simulink model "EPT"  (R2019b)
settings: Solver=FixedStepDiscrete  StartTime=0.0  StopTime=5  FixedStep=0.005  RelTol=1e-3  EnableMultiTasking=on
PreLoadFcn:
  | try, model_open; catch, disp('Error occurred while executing model pre-load callback: model_open.m'); disp('Please assure that the MATLAB working directory is set to the model directory before opening.'); end
InitFcn:
  | try, model_open; catch, end
undefined symbols (not defined in the file or in its folder): Bridge, GCM, H, ln, raptor_get_param_eval, raptor_get_safe_string, raptor_xcp_function
libraries: Raptor_lib x2810, simulink x374, hdlsllib x19
(part 8 of 45)

== system EPT/Test/LifeCycleTest/RollingCount1 ==
  In1 : Inport
  Add : Sum
  Constant3 : Constant
  Data Type Conversion : DataTypeConversion
  Data Type Conversion21 : DataTypeConversion
  NOT : Logic  Operator=NOT  IconShape=distinctive  AllPortsSameDT=off  OutDataTypeStr=boolean
  Relational Operator : RelationalOperator  Operator=>  OutDataTypeStr=boolean  RndMeth=Simplest
  Switch : Switch  Criteria=u2 > Threshold
  Unit Delay : UnitDelay  SampleTime=-1  HasFrameUpgradeWarning=on
  Out1 : Outport  VectorParamsAs1DForOutWhenUnconnected=off
  wires:
  Data Type Conversion/1 -> Out1/1
  NOT/1 -> Data Type Conversion21/1, Switch/3
  Unit Delay/1 -> Add/1
  Constant3/1 -> Add/2
  Relational Operator/1 -> NOT/1
  Add/1 -> Switch/1, Relational Operator/1
  Data Type Conversion21/1 -> Switch/2
  Switch/1 -> Data Type Conversion/1, Unit Delay/1
  In1/1 -> Relational Operator/2

== system EPT/Test/RPB1600_Read/CountTrigger ==
  Counter : Inport
  Constant1 : Constant  Value=0
  Constant3 : Constant
  CycleTrigger : Subsystem
  Switch : Switch  Threshold=1
  Unit Delay1 : UnitDelay  SampleTime=-1  HasFrameUpgradeWarning=on
  Unit Delay2 : UnitDelay  SampleTime=-1  HasFrameUpgradeWarning=on
  Tirgger : Outport  VectorParamsAs1DForOutWhenUnconnected=off
  wires:
  Unit Delay2/1 -> Tirgger/1
  Unit Delay1/1 -> CycleTrigger/1(In1)
  CycleTrigger/1(Trigger) -> Unit Delay2/1, Switch/2
  Counter/1 -> CycleTrigger/2(In2)
  Constant1/1 -> Switch/1
  Constant3/1 -> Switch/3
  Switch/1 -> Unit Delay1/1

== system EPT/Test/RPB1600_Read/RPB1600_Cmd_20ms ==
  ID : Inport
  DataBytes : Inport  Port=2
  Command : Inport  Port=3
  Trigger : TriggerPort  VariantControl=Variant  PortDimensions=1
  Add : Sum
  Constant : Constant  Value=2
  Constant1 : Constant  OutDataTypeStr=boolean
  raptor_can_txraw : Raptor_lib/CAN/raptor_can_txraw  canBus='CAN1'  queueSize=1  showIdTypePort=1  idTypeSelectValues=Standard|Extended  idTypeSelect=Standard
      settings: SourceProductName=Raptor
  wires:
  Add/1 -> raptor_can_txraw/3
  DataBytes/1 -> Add/1
  Constant/1 -> Add/2
  Constant1/1 -> raptor_can_txraw/1
  Command/1 -> raptor_can_txraw/4
  ID/1 -> raptor_can_txraw/2

== system EPT/Test/RPB1600_Read/RPB1600_RX_20ms ==
  note: 0x0000:OPERATION
      | 0x0020:VOUT_SET
      | 0x0030:IOUT_SET
      | 0x0040:FAULT_STATUS
      | 0x0050:READ_VIN
      | 0x0060:READ_VOUT
      | 0x0061:READ_IOUT
      | 0x0062:READ_TEMPERATURE_1
      | 0x0070:READ_FAN_SPEED_1
      | 0x0071:READ_FAN_SPEED_2
  Task : Inport
  "Resolution " : Inport  Port=2
  Trigger : TriggerPort  TriggerType=falling  VariantControl=Variant  PortDimensions=1
  Constant : Constant  Value=0
  Constant1 : Constant
  Constant2 : Constant  Value=2
  Constant3 : Constant  Value=3
  Constant4 : Constant  Value=4
  Constant5 : Constant  Value=5
  Constant6 : Constant  Value=6
  Constant7 : Constant  Value=7
  Constant8 : Constant  Value=8
  Constant9 : Constant  Value=9
  Convert_Byte2Data : Subsystem
  Demux : Demux  Outputs=8
  Subsystem : Subsystem
  Subsystem1 : Subsystem
  Subsystem2 : Subsystem
  Subsystem3 : Subsystem
  Subsystem4 : Subsystem
  Subsystem5 : Subsystem
  Subsystem6 : Subsystem
  Subsystem7 : Subsystem
  Subsystem8 : Subsystem
  Subsystem9 : Subsystem
  Task Rolling : Subsystem
  raptor_can_rxraw : Raptor_lib/CAN/raptor_can_rxraw  canBus='CAN1'  extendedId=1  showAge=1  id=hex2dec('C0100')  idMask=hex2dec('1FFFFFFF')  mailbox=''  queueSize=1
      settings: SourceProductName=Raptor
  raptor_measurement : Raptor_lib/Data Storage/raptor_measurement  paramName='Read_OPERATION'  nameSource=Parameter  calDispType=Number  calEnum={'False', 'True'}  calGain=1.0  calOffset=0.0  calMax=inf  calMin=-inf  calFormat='-1'  calUnit=''  calHelp=''  calAccess=1  calFunction=raptor_xcp_function(gcb)  calVisible=on
      settings: SourceProductName=Raptor
  raptor_measurement1 : Raptor_lib/Data Storage/raptor_measurement  paramName='Read_VOUT_SET'  nameSource=Parameter  calDispType=Number  calEnum={'False', 'True'}  calGain=1.0  calOffset=0.0  calMax=inf  calMin=-inf  calFormat='-1'  calUnit=''  calHelp=''  calAccess=1  calFunction=raptor_xcp_function(gcb)  calVisible=on
      settings: SourceProductName=Raptor
  raptor_measurement2 : Raptor_lib/Data Storage/raptor_measurement  paramName='Read_IOUT_SET'  nameSource=Parameter  calDispType=Number  calEnum={'False', 'True'}  calGain=1.0  calOffset=0.0  calMax=inf  calMin=-inf  calFormat='-1'  calUnit=''  calHelp=''  calAccess=1  calFunction=raptor_xcp_function(gcb)  calVisible=on
      settings: SourceProductName=Raptor
  raptor_measurement3 : Raptor_lib/Data Storage/raptor_measurement  paramName='FAULT_STATUS'  nameSource=Parameter  calDispType=Number  calEnum={'False', 'True'}  calGain=1.0  calOffset=0.0  calMax=inf  calMin=-inf  calFormat='-1'  calUnit=''  calHelp=''  calAccess=1  calFunction=raptor_xcp_function(gcb)  calVisible=on
      settings: SourceProductName=Raptor
  raptor_measurement4 : Raptor_lib/Data Storage/raptor_measurement  paramName='READ_VIN'  nameSource=Parameter  calDispType=Number  calEnum={'False', 'True'}  calGain=1.0  calOffset=0.0  calMax=inf  calMin=-inf  calFormat='-1'  calUnit=''  calHelp=''  calAccess=1  calFunction=raptor_xcp_function(gcb)  calVisible=on
      settings: SourceProductName=Raptor
  raptor_measurement5 : Raptor_lib/Data Storage/raptor_measurement  paramName='READ_VOUT'  nameSource=Parameter  calDispType=Number  calEnum={'False', 'True'}  calGain=1.0  calOffset=0.0  calMax=inf  calMin=-inf  calFormat='-1'  calUnit=''  calHelp=''  calAccess=1  calFunction=raptor_xcp_function(gcb)  calVisible=on
      settings: SourceProductName=Raptor
  raptor_measurement6 : Raptor_lib/Data Storage/raptor_measurement  paramName='READ_TEMPERATURE_1'  nameSource=Parameter  calDispType=Number  calEnum={'False', 'True'}  calGain=1.0  calOffset=0.0  calMax=inf  calMin=-inf  calFormat='-1'  calUnit=''  calHelp=''  calAccess=1  calFunction=raptor_xcp_function(gcb)  calVisible=on
      settings: SourceProductName=Raptor
  raptor_measurement7 : Raptor_lib/Data Storage/raptor_measurement  paramName='READ_IOUT'  nameSource=Parameter  calDispType=Number  calEnum={'False', 'True'}  calGain=1.0  calOffset=0.0  calMax=inf  calMin=-inf  calFormat='-1'  calUnit=''  calHelp=''  calAccess=1  calFunction=raptor_xcp_function(gcb)  calVisible=on
      settings: SourceProductName=Raptor
  raptor_measurement8 : Raptor_lib/Data Storage/raptor_measurement  paramName='READ_FAN_SPEED_1'  nameSource=Parameter  calDispType=Number  calEnum={'False', 'True'}  calGain=1.0  calOffset=0.0  calMax=inf  calMin=-inf  calFormat='-1'  calUnit=''  calHelp=''  calAccess=1  calFunction=raptor_xcp_function(gcb)  calVisible=on
      settings: SourceProductName=Raptor
  raptor_measurement9 : Raptor_lib/Data Storage/raptor_measurement  paramName='READ_FAN_SPEED_2'  nameSource=Parameter  calDispType=Number  calEnum={'False', 'True'}  calGain=1.0  calOffset=0.0  calMax=inf  calMin=-inf  calFormat='-1'  calUnit=''  calHelp=''  calAccess=1  calFunction=raptor_xcp_function(gcb)  calVisible=on
      settings: SourceProductName=Raptor
  wires:
  Task/1 -> Subsystem7/2(Task Input), Subsystem8/2(Task Input), Subsystem9/2(Task Input), Subsystem6/2(Task Input), Subsystem5/2(Task Input), Subsystem4/2(Task Input), Subsystem3/2(Task Input), Subsystem2/2(Task Input), Subsystem1/2(Task Input), Subsystem/2(Task Input)
  Constant/1 -> Subsystem/3("Task Set ")
  Constant1/1 -> Subsystem1/3("Task Set ")
  Constant2/1 -> Subsystem2/3("Task Set ")
  Constant4/1 -> Subsystem4/3("Task Set ")
  Constant5/1 -> Subsystem5/3("Task Set ")
  Constant6/1 -> Subsystem6/3("Task Set ")
  Constant7/1 -> Subsystem7/3("Task Set ")
  Constant9/1 -> Subsystem9/3("Task Set ")
  raptor_can_rxraw/5 -> Demux/1
  Demux/1 -> Convert_Byte2Data/1(LowByte)
  Demux/2 -> Convert_Byte2Data/2(HighByte)
  "Resolution "/1 -> Convert_Byte2Data/4(Factor)
  Constant3/1 -> Subsystem3/3("Task Set ")
  Constant8/1 -> Subsystem8/3("Task Set ")
  Convert_Byte2Data/1(Data(int16)) -> Subsystem9/1(Rx Data), Subsystem8/1(Rx Data), Subsystem7/1(Rx Data), Subsystem6/1(Rx Data), Subsystem5/1(Rx Data), Subsystem4/1(Rx Data), Subsystem3/1(Rx Data), Subsystem2/1(Rx Data), Subsystem1/1(Rx Data), Subsystem/1(Rx Data)
  Subsystem/1(Output) -> raptor_measurement/1
  Subsystem1/1(Output) -> raptor_measurement1/1
  Subsystem2/1(Output) -> raptor_measurement2/1
  Subsystem3/1(Output) -> raptor_measurement3/1
  Subsystem4/1(Output) -> raptor_measurement4/1
  Subsystem5/1(Output) -> raptor_measurement5/1
  Subsystem6/1(Output) -> raptor_measurement7/1
  Subsystem7/1(Output) -> raptor_measurement6/1
  Subsystem8/1(Output) -> raptor_measurement8/1
  Subsystem9/1(Output) -> raptor_measurement9/1

== system EPT/Foreground_TimeBase_5ms/CAN/CAN1_exec/BCU vs RMDA-BMS ==
  Trigger : TriggerPort  VariantControl=Variant  PortDimensions=1
  "BCU-OBU Output-CTL " : Subsystem
  BCU-OBU Output-EW Code : Subsystem
  BCU-OBU Status-OP G1 : Subsystem
  BCU-OBU Status-OP G2 : Subsystem
  BCU-OBU Status-OP G3 : Subsystem
  "BCU-OBU Status-OP G4 " : Subsystem
  "BP-OBU Enable CTL & OP Status " : Subsystem
  Compare To Constant : simulink/Logic and Bit Operations/Compare To Constant  relop===  const=0  OutDataTypeStr=boolean
  Compare To Constant1 : simulink/Logic and Bit Operations/Compare To Constant  relop===  const=10  OutDataTypeStr=boolean
  Compare To Constant2 : simulink/Logic and Bit Operations/Compare To Constant  relop===  const=20  OutDataTypeStr=boolean
  Compare To Constant3 : simulink/Logic and Bit Operations/Compare To Constant  relop===  const=30  OutDataTypeStr=boolean
  Compare To Constant4 : simulink/Logic and Bit Operations/Compare To Constant  relop===  const=40  OutDataTypeStr=boolean
  Compare To Constant5 : simulink/Logic and Bit Operations/Compare To Constant  relop===  const=50  OutDataTypeStr=boolean
  Compare To Constant6 : simulink/Logic and Bit Operations/Compare To Constant  relop===  const=60  OutDataTypeStr=boolean
  Compare To Constant7 : simulink/Logic and Bit Operations/Compare To Constant  relop===  const=70  OutDataTypeStr=boolean
  Compare To Constant8 : simulink/Logic and Bit Operations/Compare To Constant  relop===  const=80  OutDataTypeStr=boolean
  Compare To Constant9 : simulink/Logic and Bit Operations/Compare To Constant  relop===  const=90  OutDataTypeStr=boolean
  Constant2 : Constant  Value=100
  Constant3 : Constant  Value=100
  Delay{,1..8} (9 alike) : Delay
  Rem : Math  Operator=rem  SaturateOnIntegerOverflow=on
  Remote DAG2-5E0 : Subsystem
  Remote DAG2-5E1 : Subsystem
  Remote DAG2-5E2 : Subsystem
  Remote DAG2-5E3 : Subsystem
  Remote DAG2-5E4 : Subsystem
  Remote DAG2-5E5 : Subsystem
  Remote DAG2-5E6 : Subsystem
  Remote DAG2-5E7 : Subsystem
  Remote DAG2-5E8 : Subsystem
  Remote DAG2-5E9 : Subsystem
  Remote DAG2-5EA : Subsystem
  Remote DAG2-5EB : Subsystem
  RollingCount : Subsystem
  wires:
  Rem/1 -> Compare To Constant9/1, Compare To Constant8/1, Compare To Constant7/1, Compare To Constant6/1, Compare To Constant5/1, Compare To Constant4/1, Compare To Constant3/1, Compare To Constant2/1, Compare To Constant1/1, Compare To Constant/1
  Constant2/1 -> RollingCount/1(In1)
  Constant3/1 -> Rem/2
  RollingCount/1(Out1) -> Rem/1
  Compare To Constant9/1 -> Delay2/1, "BCU-OBU Status-OP G4 "/Trigger
  Compare To Constant8/1 -> BCU-OBU Status-OP G3/Trigger, Delay8/1
  Compare To Constant7/1 -> Delay7/1, BCU-OBU Status-OP G2/Trigger
  Compare To Constant6/1 -> Delay6/1, BCU-OBU Status-OP G1/Trigger
  Compare To Constant5/1 -> Delay4/1, "BCU-OBU Output-CTL "/Trigger
  Compare To Constant/1 -> Delay/1, Remote DAG2-5E0/Trigger
  Compare To Constant1/1 -> Delay1/1, Remote DAG2-5E1/Trigger
  Compare To Constant2/1 -> Delay3/1, Remote DAG2-5E2/Trigger
  Compare To Constant3/1 -> Remote DAG2-5E3/Trigger
  Compare To Constant4/1 -> Delay5/1, Remote DAG2-5E4/Trigger
  Delay/1 -> Remote DAG2-5E9/Trigger
  Delay1/1 -> Remote DAG2-5EA/Trigger
  Delay6/1 -> Remote DAG2-5E5/Trigger
  Delay7/1 -> Remote DAG2-5E6/Trigger
  Delay8/1 -> Remote DAG2-5E7/Trigger
  Delay2/1 -> Remote DAG2-5E8/Trigger
  Delay3/1 -> Remote DAG2-5EB/Trigger
  Delay4/1 -> BCU-OBU Output-EW Code/Trigger
  Delay5/1 -> "BP-OBU Enable CTL & OP Status "/Trigger

== system EPT/Foreground_TimeBase_5ms/CAN/CAN1_exec/BCU-CMU ==
  Enable : EnablePort
  CMU_Task : Subsystem

== system EPT/Foreground_TimeBase_5ms/CAN/CAN1_exec/CountTrigger1 ==
  Counter : Inport
  Constant1 : Constant  Value=0
  Constant3 : Constant
  CycleTrigger : Subsystem
  Switch : Switch  Threshold=1
  Unit Delay1 : UnitDelay  SampleTime=-1  HasFrameUpgradeWarning=on
  Unit Delay2 : UnitDelay  SampleTime=-1  HasFrameUpgradeWarning=on
  Tirgger : Outport  VectorParamsAs1DForOutWhenUnconnected=off
  wires:
  Switch/1 -> Unit Delay1/1
  Constant3/1 -> Switch/3
  Constant1/1 -> Switch/1
  Counter/1 -> CycleTrigger/2(In2)
  CycleTrigger/1(Trigger) -> Switch/2, Unit Delay2/1
  Unit Delay1/1 -> CycleTrigger/1(In1)
  Unit Delay2/1 -> Tirgger/1

== system EPT/Foreground_TimeBase_5ms/CAN/CAN1_exec/IVT ==
  Enable : EnablePort
  Constant1 : Constant  Value=4
  Constant2 : Constant  Value=12
  CountTrigger : Subsystem
  CountTrigger1 : Subsystem
  Delay : Delay  DelayLength=1
  "IVT_RX_0x521 " : Subsystem  TreatAsAtomicUnit=on
  IVT_RX_0x522 : Subsystem  TreatAsAtomicUnit=on
  IVT_RX_0x523 : Subsystem  TreatAsAtomicUnit=on
  IVT_RX_0x524 : Subsystem  TreatAsAtomicUnit=on
  wires:
  Delay/1 -> IVT_RX_0x523/Trigger, IVT_RX_0x524/Trigger
  Constant2/1 -> CountTrigger1/1(Counter)
  CountTrigger1/1(Tirgger) -> IVT_RX_0x522/Trigger, Delay/1
  CountTrigger/1(Tirgger) -> "IVT_RX_0x521 "/Trigger
  Constant1/1 -> CountTrigger/1(Counter)

== system EPT/Foreground_TimeBase_5ms/CAN/CAN2_exec/BCU vs ITRI//ARTC ==
  Enable : EnablePort
  "BCU-OBU Output-CTL " : Subsystem
  BCU-OBU Output-EW Code : Subsystem
  BCU-OBU Status-OP G1 : Subsystem
  BCU-OBU Status-OP G2 : Subsystem
  BCU-OBU Status-OP G3 : Subsystem
  "BCU-OBU Status-OP G4 " : Subsystem
  "BP-OBU Enable CTL & OP Status " : Subsystem
  CountTrigger1 : Subsystem
  Delay{,1..17} (18 alike) : Delay  DelayLength=1  InitialCondition=0  UseCircularBuffer=on
  Remote DAG2-5E0 : Subsystem
  Remote DAG2-5E1 : Subsystem
  Remote DAG2-5E2 : Subsystem
  Remote DAG2-5E3 : Subsystem
  Remote DAG2-5E4 : Subsystem
  Remote DAG2-5E5 : Subsystem
  Remote DAG2-5E6 : Subsystem
  Remote DAG2-5E7 : Subsystem
  Remote DAG2-5E8 : Subsystem
  Remote DAG2-5E9 : Subsystem
  Remote DAG2-5EA : Subsystem
  Remote DAG2-5EB : Subsystem
  raptor_adjustment : Raptor_lib/Data Storage/raptor_adjustment  paramName='Cal_CAN2ITRI_TxTime'  nameSource=Parameter  initValue=100  dataType=double  storage=Calibration  calDispType=Number  calEnum={'False', 'True'}  calGain=1.0  calOffset=0.0  calMax=inf  calMin=-inf  calFormat='-1'  calUnit=''  calHelp=''  calAccess=1  calFunction=raptor_xcp_function(gcb)  calDispHeaders=off  calColHeaders={'Col1' 'Col2' 'Col3'}  calRowHeaders={'Row1' 'Row2' 'Row3'}
      settings: SourceProductName=Raptor
  raptor_adjustment1 : Raptor_lib/Data Storage/raptor_adjustment  paramName='Cal_BCU_OBU_Status_OP_G1_CANon'  nameSource=Parameter  initValue=0.00  dataType=double  storage=Calibration  calDispType=Number  calEnum={'False', 'True'}  calGain=1.0  calOffset=0.0  calMax=inf  calMin=-inf  calFormat='-1'  calUnit=''  calHelp=''  calAccess=1  calFunction=raptor_xcp_function(gcb)  calDispHeaders=off  calColHeaders={'Col1' 'Col2' 'Col3'}  calRowHeaders={'Row1' 'Row2' 'Row3'}
      settings: SourceProductName=Raptor
  raptor_adjustment10 : Raptor_lib/Data Storage/raptor_adjustment  paramName='Cal_BCU_OBU_DAG2_5E7_CANon'  nameSource=Parameter  initValue=0.00  dataType=double  storage=Calibration  calDispType=Number  calEnum={'False', 'True'}  calGain=1.0  calOffset=0.0  calMax=inf  calMin=-inf  calFormat='-1'  calUnit=''  calHelp=''  calAccess=1  calFunction=raptor_xcp_function(gcb)  calDispHeaders=off  calColHeaders={'Col1' 'Col2' 'Col3'}  calRowHeaders={'Row1' 'Row2' 'Row3'}
      settings: SourceProductName=Raptor
  raptor_adjustment11 : Raptor_lib/Data Storage/raptor_adjustment  paramName='Cal_BCU_OBU_DAG2_5E8_CANon'  nameSource=Parameter  initValue=0.00  dataType=double  storage=Calibration  calDispType=Number  calEnum={'False', 'True'}  calGain=1.0  calOffset=0.0  calMax=inf  calMin=-inf  calFormat='-1'  calUnit=''  calHelp=''  calAccess=1  calFunction=raptor_xcp_function(gcb)  calDispHeaders=off  calColHeaders={'Col1' 'Col2' 'Col3'}  calRowHeaders={'Row1' 'Row2' 'Row3'}
      settings: SourceProductName=Raptor
  raptor_adjustment12 : Raptor_lib/Data Storage/raptor_adjustment  paramName='Cal_BCU_OBU_DAG2_5EB_CANon'  nameSource=Parameter  initValue=0.00  dataType=double  storage=Calibration  calDispType=Number  calEnum={'False', 'True'}  calGain=1.0  calOffset=0.0  calMax=inf  calMin=-inf  calFormat='-1'  calUnit=''  calHelp=''  calAccess=1  calFunction=raptor_xcp_function(gcb)  calDispHeaders=off  calColHeaders={'Col1' 'Col2' 'Col3'}  calRowHeaders={'Row1' 'Row2' 'Row3'}
      settings: SourceProductName=Raptor
  raptor_adjustment13 : Raptor_lib/Data Storage/raptor_adjustment  paramName='Cal_BCU_OBU_DAG2_5E9_CANon'  nameSource=Parameter  initValue=0.00  dataType=double  storage=Calibration  calDispType=Number  calEnum={'False', 'True'}  calGain=1.0  calOffset=0.0  calMax=inf  calMin=-inf  calFormat='-1'  calUnit=''  calHelp=''  calAccess=1  calFunction=raptor_xcp_function(gcb)  calDispHeaders=off  calColHeaders={'Col1' 'Col2' 'Col3'}  calRowHeaders={'Row1' 'Row2' 'Row3'}
      settings: SourceProductName=Raptor
  raptor_adjustment14 : Raptor_lib/Data Storage/raptor_adjustment  paramName='Cal_BCU_OBU_DAG2_5EA_CANon'  nameSource=Parameter  initValue=0.00  dataType=double  storage=Calibration  calDispType=Number  calEnum={'False', 'True'}  calGain=1.0  calOffset=0.0  calMax=inf  calMin=-inf  calFormat='-1'  calUnit=''  calHelp=''  calAccess=1  calFunction=raptor_xcp_function(gcb)  calDispHeaders=off  calColHeaders={'Col1' 'Col2' 'Col3'}  calRowHeaders={'Row1' 'Row2' 'Row3'}
      settings: SourceProductName=Raptor
  raptor_adjustment15 : Raptor_lib/Data Storage/raptor_adjustment  paramName='Cal_BCU_OBU_DAG2_5E3_CANon'  nameSource=Parameter  initValue=0.00  dataType=double  storage=Calibration  calDispType=Number  calEnum={'False', 'True'}  calGain=1.0  calOffset=0.0  calMax=inf  calMin=-inf  calFormat='-1'  calUnit=''  calHelp=''  calAccess=1  calFunction=raptor_xcp_function(gcb)  calDispHeaders=off  calColHeaders={'Col1' 'Col2' 'Col3'}  calRowHeaders={'Row1' 'Row2' 'Row3'}
      settings: SourceProductName=Raptor
  raptor_adjustment16 : Raptor_lib/Data Storage/raptor_adjustment  paramName='Cal_BCU_OBU_DAG2_5E4_CANon'  nameSource=Parameter  initValue=0.00  dataType=double  storage=Calibration  calDispType=Number  calEnum={'False', 'True'}  calGain=1.0  calOffset=0.0  calMax=inf  calMin=-inf  calFormat='-1'  calUnit=''  calHelp=''  calAccess=1  calFunction=raptor_xcp_function(gcb)  calDispHeaders=off  calColHeaders={'Col1' 'Col2' 'Col3'}  calRowHeaders={'Row1' 'Row2' 'Row3'}
      settings: SourceProductName=Raptor
  raptor_adjustment17 : Raptor_lib/Data Storage/raptor_adjustment  paramName='Cal_BCU_OBU_DAG2_5E0_CANon'  nameSource=Parameter  initValue=0.00  dataType=double  storage=Calibration  calDispType=Number  calEnum={'False', 'True'}  calGain=1.0  calOffset=0.0  calMax=inf  calMin=-inf  calFormat='-1'  calUnit=''  calHelp=''  calAccess=1  calFunction=raptor_xcp_function(gcb)  calDispHeaders=off  calColHeaders={'Col1' 'Col2' 'Col3'}  calRowHeaders={'Row1' 'Row2' 'Row3'}
      settings: SourceProductName=Raptor
  raptor_adjustment2 : Raptor_lib/Data Storage/raptor_adjustment  paramName='Cal_BCU_OBU_Status_OP_G2_CANon'  nameSource=Parameter  initValue=0.00  dataType=double  storage=Calibration  calDispType=Number  calEnum={'False', 'True'}  calGain=1.0  calOffset=0.0  calMax=inf  calMin=-inf  calFormat='-1'  calUnit=''  calHelp=''  calAccess=1  calFunction=raptor_xcp_function(gcb)  calDispHeaders=off  calColHeaders={'Col1' 'Col2' 'Col3'}  calRowHeaders={'Row1' 'Row2' 'Row3'}
      settings: SourceProductName=Raptor
  raptor_adjustment20 : Raptor_lib/Data Storage/raptor_adjustment  paramName='Cal_BCU_OBU_DAG2_5E1_CANon'  nameSource=Parameter  initValue=0.00  dataType=double  storage=Calibration  calDispType=Number  calEnum={'False', 'True'}  calGain=1.0  calOffset=0.0  calMax=inf  calMin=-inf  calFormat='-1'  calUnit=''  calHelp=''  calAccess=1  calFunction=raptor_xcp_function(gcb)  calDispHeaders=off  calColHeaders={'Col1' 'Col2' 'Col3'}  calRowHeaders={'Row1' 'Row2' 'Row3'}
      settings: SourceProductName=Raptor
  raptor_adjustment21 : Raptor_lib/Data Storage/raptor_adjustment  paramName='Cal_BCU_OBU_DAG2_5E2_CANon'  nameSource=Parameter  initValue=0.00  dataType=double  storage=Calibration  calDispType=Number  calEnum={'False', 'True'}  calGain=1.0  calOffset=0.0  calMax=inf  calMin=-inf  calFormat='-1'  calUnit=''  calHelp=''  calAccess=1  calFunction=raptor_xcp_function(gcb)  calDispHeaders=off  calColHeaders={'Col1' 'Col2' 'Col3'}  calRowHeaders={'Row1' 'Row2' 'Row3'}
      settings: SourceProductName=Raptor
  raptor_adjustment3 : Raptor_lib/Data Storage/raptor_adjustment  paramName='Cal_BCU_OBU_Status_OP_G3_CANon'  nameSource=Parameter  initValue=0.00  dataType=double  storage=Calibration  calDispType=Number  calEnum={'False', 'True'}  calGain=1.0  calOffset=0.0  calMax=inf  calMin=-inf  calFormat='-1'  calUnit=''  calHelp=''  calAccess=1  calFunction=raptor_xcp_function(gcb)  calDispHeaders=off  calColHeaders={'Col1' 'Col2' 'Col3'}  calRowHeaders={'Row1' 'Row2' 'Row3'}
      settings: SourceProductName=Raptor
  raptor_adjustment4 : Raptor_lib/Data Storage/raptor_adjustment  paramName='Cal_BCU_OBU_Status_OP_G4_CANon'  nameSource=Parameter  initValue=0.00  dataType=double  storage=Calibration  calDispType=Number  calEnum={'False', 'True'}  calGain=1.0  calOffset=0.0  calMax=inf  calMin=-inf  calFormat='-1'  calUnit=''  calHelp=''  calAccess=1  calFunction=raptor_xcp_function(gcb)  calDispHeaders=off  calColHeaders={'Col1' 'Col2' 'Col3'}  calRowHeaders={'Row1' 'Row2' 'Row3'}
      settings: SourceProductName=Raptor
  raptor_adjustment5 : Raptor_lib/Data Storage/raptor_adjustment  paramName='Cal_BCU_OBU_Output_CTL_CANon'  nameSource=Parameter  initValue=0.00  dataType=double  storage=Calibration  calDispType=Number  calEnum={'False', 'True'}  calGain=1.0  calOffset=0.0  calMax=inf  calMin=-inf  calFormat='-1'  calUnit=''  calHelp=''  calAccess=1  calFunction=raptor_xcp_function(gcb)  calDispHeaders=off  calColHeaders={'Col1' 'Col2' 'Col3'}  calRowHeaders={'Row1' 'Row2' 'Row3'}
      settings: SourceProductName=Raptor
  raptor_adjustment6 : Raptor_lib/Data Storage/raptor_adjustment  paramName='Cal_BCU_OBU_Enable_CTL_OP_tatus_CANon'  nameSource=Parameter  initValue=0.00  dataType=double  storage=Calibration  calDispType=Number  calEnum={'False', 'True'}  calGain=1.0  calOffset=0.0  calMax=inf  calMin=-inf  calFormat='-1'  calUnit=''  calHelp=''  calAccess=1  calFunction=raptor_xcp_function(gcb)  calDispHeaders=off  calColHeaders={'Col1' 'Col2' 'Col3'}  calRowHeaders={'Row1' 'Row2' 'Row3'}
      settings: SourceProductName=Raptor
  raptor_adjustment7 : Raptor_lib/Data Storage/raptor_adjustment  paramName='Cal_BCU_OBU_Output_EW_Code_CANon'  nameSource=Parameter  initValue=0.00  dataType=double  storage=Calibration  calDispType=Number  calEnum={'False', 'True'}  calGain=1.0  calOffset=0.0  calMax=inf  calMin=-inf  calFormat='-1'  calUnit=''  calHelp=''  calAccess=1  calFunction=raptor_xcp_function(gcb)  calDispHeaders=off  calColHeaders={'Col1' 'Col2' 'Col3'}  calRowHeaders={'Row1' 'Row2' 'Row3'}
      settings: SourceProductName=Raptor
  raptor_adjustment8 : Raptor_lib/Data Storage/raptor_adjustment  paramName='Cal_BCU_OBU_DAG2_5E5_CANon'  nameSource=Parameter  initValue=0.00  dataType=double  storage=Calibration  calDispType=Number  calEnum={'False', 'True'}  calGain=1.0  calOffset=0.0  calMax=inf  calMin=-inf  calFormat='-1'  calUnit=''  calHelp=''  calAccess=1  calFunction=raptor_xcp_function(gcb)  calDispHeaders=off  calColHeaders={'Col1' 'Col2' 'Col3'}  calRowHeaders={'Row1' 'Row2' 'Row3'}
      settings: SourceProductName=Raptor
  raptor_adjustment9 : Raptor_lib/Data Storage/raptor_adjustment  paramName='Cal_BCU_OBU_DAG2_5E6_CANon'  nameSource=Parameter  initValue=0.00  dataType=double  storage=Calibration  calDispType=Number  calEnum={'False', 'True'}  calGain=1.0  calOffset=0.0  calMax=inf  calMin=-inf  calFormat='-1'  calUnit=''  calHelp=''  calAccess=1  calFunction=raptor_xcp_function(gcb)  calDispHeaders=off  calColHeaders={'Col1' 'Col2' 'Col3'}  calRowHeaders={'Row1' 'Row2' 'Row3'}
      settings: SourceProductName=Raptor
  wires:
  CountTrigger1/1(Tirgger) -> Delay17/1, Remote DAG2-5E0/Trigger
  Delay/1 -> Delay1/1, Remote DAG2-5E2/Trigger
  Delay1/1 -> Delay2/1, Remote DAG2-5E3/Trigger
  Delay2/1 -> Delay3/1, Remote DAG2-5E4/Trigger
  Delay3/1 -> Delay4/1, Remote DAG2-5E8/Trigger
  Delay4/1 -> Delay5/1, Remote DAG2-5E7/Trigger
  Delay5/1 -> Delay6/1, Remote DAG2-5E6/Trigger
  Delay6/1 -> Delay7/1, Remote DAG2-5E5/Trigger
  Delay7/1 -> Delay8/1, Remote DAG2-5E9/Trigger
  Delay8/1 -> Delay9/1, Remote DAG2-5EA/Trigger
  Delay9/1 -> Delay10/1, Remote DAG2-5EB/Trigger
  Delay10/1 -> Delay11/1, "BCU-OBU Status-OP G4 "/Trigger
  Delay11/1 -> Delay12/1, BCU-OBU Status-OP G3/Trigger
  Delay12/1 -> Delay13/1, BCU-OBU Status-OP G2/Trigger
  Delay13/1 -> BCU-OBU Status-OP G1/Trigger, Delay14/1
  Delay14/1 -> Delay15/1, "BCU-OBU Output-CTL "/Trigger
  Delay15/1 -> Delay16/1, "BP-OBU Enable CTL & OP Status "/Trigger
  Delay16/1 -> BCU-OBU Output-EW Code/Trigger
  raptor_adjustment/1 -> CountTrigger1/1(Counter)
  raptor_adjustment1/1 -> BCU-OBU Status-OP G1/Enable
  raptor_adjustment2/1 -> BCU-OBU Status-OP G2/Enable
  raptor_adjustment3/1 -> BCU-OBU Status-OP G3/Enable
  raptor_adjustment4/1 -> "BCU-OBU Status-OP G4 "/Enable
  raptor_adjustment5/1 -> "BCU-OBU Output-CTL "/Enable
  raptor_adjustment6/1 -> "BP-OBU Enable CTL & OP Status "/Enable
  raptor_adjustment7/1 -> BCU-OBU Output-EW Code/Enable
  raptor_adjustment13/1 -> Remote DAG2-5E9/Enable
  raptor_adjustment14/1 -> Remote DAG2-5EA/Enable
  raptor_adjustment12/1 -> Remote DAG2-5EB/Enable
  raptor_adjustment10/1 -> Remote DAG2-5E7/Enable
  raptor_adjustment11/1 -> Remote DAG2-5E8/Enable
  raptor_adjustment9/1 -> Remote DAG2-5E6/Enable
  raptor_adjustment8/1 -> Remote DAG2-5E5/Enable
  raptor_adjustment16/1 -> Remote DAG2-5E4/Enable
  raptor_adjustment15/1 -> Remote DAG2-5E3/Enable
  raptor_adjustment21/1 -> Remote DAG2-5E2/Enable
  raptor_adjustment20/1 -> Remote DAG2-5E1/Enable
  raptor_adjustment17/1 -> Remote DAG2-5E0/Enable
  Delay17/1 -> Remote DAG2-5E1/Trigger, Delay/1

== system EPT/Foreground_TimeBase_5ms/CAN/CAN2_exec/ECHS ==
  Enable : EnablePort
  Constant1 : Constant  Value=2
  CountTrigger : Subsystem
  EPT2ECHS_RX : Subsystem  TreatAsAtomicUnit=on
  EPT2ECHS_TX : Subsystem  TreatAsAtomicUnit=on
  wires:
  CountTrigger/1(Tirgger) -> EPT2ECHS_TX/Trigger, EPT2ECHS_RX/Trigger
  Constant1/1 -> CountTrigger/1(Counter)

== system EPT/Foreground_TimeBase_5ms/CAN/CAN2_exec/IVT2 ==
  Constant1 : Constant  Value=4
  Constant2 : Constant  Value=12
  Coulomb Counting Method1 : Subsystem
  CountTrigger : Subsystem
  CountTrigger1 : Subsystem
  Delay : Delay  DelayLength=1
  Delay1 : Delay  DelayLength=1
  Delay2 : Subsystem
  Delay3 : Subsystem
  Divide : Product  Inputs=*/
  Gain : Gain  Gain=100
  Gain1 : Gain  Gain=-1
  "IVT_RX_0x521 " : Subsystem  TreatAsAtomicUnit=on
  IVT_RX_0x522 : Subsystem  TreatAsAtomicUnit=on
  IVT_RX_0x523 : Subsystem  TreatAsAtomicUnit=on
  IVT_RX_0x524 : Subsystem  TreatAsAtomicUnit=on
  Latch : Subsystem
  Latch1 : Subsystem
  Logical Operator : Logic  Inputs=4  AllPortsSameDT=off  OutDataTypeStr=boolean
  NOT : Logic  Operator=NOT  IconShape=distinctive  AllPortsSameDT=off  OutDataTypeStr=boolean
  NOT1 : Logic  Operator=NOT  IconShape=distinctive  AllPortsSameDT=off  OutDataTypeStr=boolean
  NOT2 : Logic  Operator=NOT  IconShape=distinctive  AllPortsSameDT=off  OutDataTypeStr=boolean
  Relational Operator : RelationalOperator  OutDataTypeStr=boolean  RndMeth=Simplest
  Relational Operator1 : RelationalOperator  Operator=<=  OutDataTypeStr=boolean  RndMeth=Simplest
  Relational Operator2 : RelationalOperator  Operator=<=  OutDataTypeStr=boolean  RndMeth=Simplest
  raptor_adjustment : Raptor_lib/Data Storage/raptor_adjustment  paramName='Cal_BatteryCell_AHmax'  nameSource=Parameter  initValue=50  dataType=double  storage=Calibration  calDispType=Number  calEnum={'False', 'True'}  calGain=1.0  calOffset=0.0  calMax=inf  calMin=-inf  calFormat='-1'  calUnit=''  calHelp=''  calAccess=1  calFunction=raptor_xcp_function(gcb)  calDispHeaders=off  calColHeaders={'Col1' 'Col2' 'Col3'}  calRowHeaders={'Row1' 'Row2' 'Row3'}
      settings: SourceProductName=Raptor
  raptor_adjustment1 : Raptor_lib/Data Storage/raptor_adjustment  paramName='Cal_BatteryCell_EOC_Timecount'  nameSource=Parameter  initValue=300  dataType=double  storage=Calibration  calDispType=Number  calEnum={'False', 'True'}  calGain=1.0  calOffset=0.0  calMax=inf  calMin=-inf  calFormat='-1'  calUnit=''  calHelp=''  calAccess=1  calFunction=raptor_xcp_function(gcb)  calDispHeaders=off  calColHeaders={'Col1' 'Col2' 'Col3'}  calRowHeaders={'Row1' 'Row2' 'Row3'}
      settings: SourceProductName=Raptor
  raptor_adjustment2 : Raptor_lib/Data Storage/raptor_adjustment  paramName='Cal_BatteryCell_Relay_Reset'  nameSource=Parameter  initValue=0  dataType=boolean  storage=Calibration  calDispType=Number  calEnum={'False', 'True'}  calGain=1.0  calOffset=0.0  calMax=inf  calMin=-inf  calFormat='-1'  calUnit=''  calHelp=''  calAccess=1  calFunction=raptor_xcp_function(gcb)  calDispHeaders=off  calColHeaders={'Col1' 'Col2' 'Col3'}  calRowHeaders={'Row1' 'Row2' 'Row3'}
      settings: SourceProductName=Raptor
  raptor_adjustment3 : Raptor_lib/Data Storage/raptor_adjustment  paramName='Cal_BatteryCell_CHG_DCHG_mode'  nameSource=Parameter  initValue=0  dataType=boolean  storage=Calibration  calDispType=Number  calEnum={'False', 'True'}  calGain=1.0  calOffset=0.0  calMax=inf  calMin=-inf  calFormat='-1'  calUnit=''  calHelp=''  calAccess=1  calFunction=raptor_xcp_function(gcb)  calDispHeaders=off  calColHeaders={'Col1' 'Col2' 'Col3'}  calRowHeaders={'Row1' 'Row2' 'Row3'}
      settings: SourceProductName=Raptor
  raptor_adjustment4 : Raptor_lib/Data Storage/raptor_adjustment  paramName='Cal_BatteryCell_EOC_Voltage'  nameSource=Parameter  initValue=3.56  dataType=double  storage=Calibration  calDispType=Number  calEnum={'False', 'True'}  calGain=1.0  calOffset=0.0  calMax=inf  calMin=-inf  calFormat='-1'  calUnit=''  calHelp=''  calAccess=1  calFunction=raptor_xcp_function(gcb)  calDispHeaders=off  calColHeaders={'Col1' 'Col2' 'Col3'}  calRowHeaders={'Row1' 'Row2' 'Row3'}
      settings: SourceProductName=Raptor
  raptor_adjustment5 : Raptor_lib/Data Storage/raptor_adjustment  paramName='Cal_BatteryCell_EOD_Voltage'  nameSource=Parameter  initValue=2.6  dataType=double  storage=Calibration  calDispType=Number  calEnum={'False', 'True'}  calGain=1.0  calOffset=0.0  calMax=inf  calMin=-inf  calFormat='-1'  calUnit=''  calHelp=''  calAccess=1  calFunction=raptor_xcp_function(gcb)  calDispHeaders=off  calColHeaders={'Col1' 'Col2' 'Col3'}  calRowHeaders={'Row1' 'Row2' 'Row3'}
      settings: SourceProductName=Raptor
  raptor_adjustment6 : Raptor_lib/Data Storage/raptor_adjustment  paramName='Cal_BatteryCell_EOD_Timecount'  nameSource=Parameter  initValue=300  dataType=double  storage=Calibration  calDispType=Number  calEnum={'False', 'True'}  calGain=1.0  calOffset=0.0  calMax=inf  calMin=-inf  calFormat='-1'  calUnit=''  calHelp=''  calAccess=1  calFunction=raptor_xcp_function(gcb)  calDispHeaders=off  calColHeaders={'Col1' 'Col2' 'Col3'}  calRowHeaders={'Row1' 'Row2' 'Row3'}
      settings: SourceProductName=Raptor
  raptor_adjustment7 : Raptor_lib/Data Storage/raptor_adjustment  paramName='Cal_RSOC_Condition'  nameSource=Parameter  initValue=50  dataType=double  storage=Calibration  calDispType=Number  calEnum={'False', 'True'}  calGain=1.0  calOffset=0.0  calMax=inf  calMin=-inf  calFormat='-1'  calUnit=''  calHelp=''  calAccess=1  calFunction=raptor_xcp_function(gcb)  calDispHeaders=off  calColHeaders={'Col1' 'Col2' 'Col3'}  calRowHeaders={'Row1' 'Row2' 'Row3'}
      settings: SourceProductName=Raptor
  raptor_data_write : Raptor_lib/Data Storage/raptor_data_write  dataName='K57_LSD_WakeUp_Reserved'  dataShape=Scalar  idxSource=Input Port  idxRow=1  idxCol=1
      settings: SourceProductName=Raptor
  raptor_measurement : Raptor_lib/Data Storage/raptor_measurement  paramName='BatteryCell_RC'  nameSource=Parameter  calDispType=Number  calEnum={'False', 'True'}  calGain=1.0  calOffset=0.0  calMax=inf  calMin=-inf  calFormat='-1'  calUnit=''  calHelp=''  calAccess=1  calFunction=raptor_xcp_function(gcb)  calVisible=on
      settings: SourceProductName=Raptor
  raptor_measurement1 : Raptor_lib/Data Storage/raptor_measurement  paramName='BatteryCell_RSOC'  nameSource=Parameter  calDispType=Number  calEnum={'False', 'True'}  calGain=1.0  calOffset=0.0  calMax=inf  calMin=-inf  calFormat='-1'  calUnit=''  calHelp=''  calAccess=1  calFunction=raptor_xcp_function(gcb)  calVisible=on
      settings: SourceProductName=Raptor
  raptor_override : Raptor_lib/Data Storage/raptor_override  paramName='Cal_BatteryCell_RC'  nameSource=Parameter  measurement=None  calDispType=Number  calEnum={'False', 'True'}  calGain=1.0  calOffset=0.0  calMax=inf  calMin=-inf  calFormat='-1'  calUnit=''  calHelp=''  calAccess=1  calFunction=[raptor_xcp_function(gcb) '|' raptor_get_param_eval(gcb, 'paramName') '_Override']
      settings: SourceProductName=Raptor
  wires:
  Delay/1 -> IVT_RX_0x523/Trigger, IVT_RX_0x524/Trigger
  Constant2/1 -> CountTrigger1/1(Counter)
  CountTrigger1/1(Tirgger) -> IVT_RX_0x522/Trigger, Delay/1
  CountTrigger/1(Tirgger) -> "IVT_RX_0x521 "/Trigger
  Constant1/1 -> CountTrigger/1(Counter)
  "IVT_RX_0x521 "/1(Current) -> Gain1/1
  Coulomb Counting Method1/1(RC Output) -> raptor_override/1
  Delay1/1 -> Coulomb Counting Method1/2(RC input)
  raptor_adjustment/1 -> Divide/2
  Divide/1 -> Gain/1
  Gain/1 -> Relational Operator2/1, raptor_measurement1/1
  raptor_override/1 -> Delay1/1, Divide/1, raptor_measurement/1
  Gain1/1 -> Coulomb Counting Method1/1(Ampere input)
  IVT_RX_0x522/1(U1_Voltage) -> Relational Operator1/1, Relational Operator/1
  Delay2/1(Output) -> Latch/1(Latch)
  Relational Operator/1 -> Delay2/1(Condition)
  Latch/1(Output) -> NOT/1
  raptor_adjustment1/1 -> Delay2/2(TimeCount)
  raptor_adjustment2/1 -> Latch/2(Reset), Latch1/2(Reset)
  NOT/1 -> Logical Operator/2
  raptor_adjustment3/1 -> Logical Operator/3
  Logical Operator/1 -> raptor_data_write/1
  raptor_adjustment4/1 -> Relational Operator/2
  raptor_adjustment5/1 -> Relational Operator1/2
  NOT1/1 -> Logical Operator/4
  Latch1/1(Output) -> NOT1/1
  Delay3/1(Output) -> Latch1/1(Latch)
  Relational Operator1/1 -> Delay3/1(Condition)
  raptor_adjustment6/1 -> Delay3/2(TimeCount)
  raptor_adjustment7/1 -> Relational Operator2/2
  Relational Operator2/1 -> NOT2/1
  NOT2/1 -> Logical Operator/1

== system EPT/Foreground_TimeBase_5ms/CAN/CAN2_exec/Remote DA  ==
  Enable : EnablePort
  Constant1 : Constant  Value=40
  CountTrigger : Subsystem
  Delay{,1..4,6..8} (8 alike) : Delay  DelayLength=1  InitialCondition=0
  Remote DA Status G13 (Vehicle-EPT_OP_Status#1) : Subsystem  TreatAsAtomicUnit=on
  Remote DA Status G14 (Vehicle-EPT_OP_Status#2) : Subsystem  TreatAsAtomicUnit=on
  Remote DA Status G21 (ESS-OBU#2) : Subsystem  TreatAsAtomicUnit=on
  Remote DA Status G22 (ESS-OBU#3) : Subsystem  TreatAsAtomicUnit=on
  Remote DA Status G23 (CHGer) : Subsystem  TreatAsAtomicUnit=on
  Remote DA Status G30 (ESS-SWCU) : Subsystem  TreatAsAtomicUnit=on
  Remote DA Status G31 (ESS-SWUBP#1) : Subsystem  TreatAsAtomicUnit=on
  Remote DA Status G32 (ESS-SWUBP#2) : Subsystem  TreatAsAtomicUnit=on
  Remote DA Status G33 (ESS-SWUBP#3) : Subsystem  TreatAsAtomicUnit=on
  wires:
  Constant1/1 -> CountTrigger/1(Counter)
  CountTrigger/1(Tirgger) -> Delay/1, Remote DA Status G13 (Vehicle-EPT_OP_Status#1)/Trigger
  Delay/1 -> Delay1/1, Remote DA Status G14 (Vehicle-EPT_OP_Status#2)/Trigger
  Delay1/1 -> Delay2/1, Remote DA Status G23 (CHGer)/Trigger
  Delay2/1 -> Delay3/1, Remote DA Status G22 (ESS-OBU#3)/Trigger
  Delay3/1 -> Delay4/1, Remote DA Status G21 (ESS-OBU#2)/Trigger
  Delay4/1 -> Delay6/1, Remote DA Status G30 (ESS-SWCU)/Trigger
  Delay6/1 -> Remote DA Status G31 (ESS-SWUBP#1)/Trigger, Delay7/1
  Delay7/1 -> Remote DA Status G32 (ESS-SWUBP#2)/Trigger, Delay8/1
  Delay8/1 -> Remote DA Status G33 (ESS-SWUBP#3)/Trigger

== system EPT/Foreground_TimeBase_5ms/CAN/CAN3_exec/20CH_TCS ==
  Enable : EnablePort
  CH13_CH16_Rx : Subsystem
  CH17_CH20_Rx1 : Subsystem
  CH1_CH4_Rx : Subsystem
  CH5_CH8_Rx : Subsystem
  CH9_CH12_Rx : Subsystem
  CountTrigger : Subsystem
  Delay{1..4} (4 alike) : Delay  DelayLength=1
  raptor_adjustment : Raptor_lib/Data Storage/raptor_adjustment  paramName='Cal_20CH_TCS_Factor'  nameSource=Parameter  initValue=0.03125  dataType=double  storage=Calibration  calDispType=Number  calEnum={'False', 'True'}  calGain=1.0  calOffset=0.0  calMax=inf  calMin=-inf  calFormat='-1'  calUnit=''  calHelp=''  calAccess=1  calFunction=raptor_xcp_function(gcb)  calDispHeaders=off  calColHeaders={'Col1' 'Col2' 'Col3'}  calRowHeaders={'Row1' 'Row2' 'Row3'}
      settings: SourceProductName=Raptor
  raptor_adjustment1 : Raptor_lib/Data Storage/raptor_adjustment  paramName='Cal_20CH_TCS_Offset'  nameSource=Parameter  initValue=-274  dataType=double  storage=Calibration  calDispType=Number  calEnum={'False', 'True'}  calGain=1.0  calOffset=0.0  calMax=inf  calMin=-inf  calFormat='-1'  calUnit=''  calHelp=''  calAccess=1  calFunction=raptor_xcp_function(gcb)  calDispHeaders=off  calColHeaders={'Col1' 'Col2' 'Col3'}  calRowHeaders={'Row1' 'Row2' 'Row3'}
      settings: SourceProductName=Raptor
  raptor_adjustment2 : Raptor_lib/Data Storage/raptor_adjustment  paramName='Cal_20CH_TCS_Rx_Time'  nameSource=Parameter  initValue=200  dataType=double  storage=Calibration  calDispType=Number  calEnum={'False', 'True'}  calGain=1.0  calOffset=0.0  calMax=inf  calMin=-inf  calFormat='-1'  calUnit=''  calHelp=''  calAccess=1  calFunction=raptor_xcp_function(gcb)  calDispHeaders=off  calColHeaders={'Col1' 'Col2' 'Col3'}  calRowHeaders={'Row1' 'Row2' 'Row3'}
      settings: SourceProductName=Raptor
  wires:
  raptor_adjustment2/1 -> CountTrigger/1(Counter)
  CountTrigger/1(Tirgger) -> CH1_CH4_Rx/Trigger, Delay2/1
  Delay2/1 -> Delay1/1, CH5_CH8_Rx/Trigger
  Delay1/1 -> Delay3/1, CH9_CH12_Rx/Trigger
  Delay4/1 -> CH17_CH20_Rx1/Trigger
  Delay3/1 -> Delay4/1, CH13_CH16_Rx/Trigger
  raptor_adjustment/1 -> CH1_CH4_Rx/1(Factor), CH17_CH20_Rx1/1(Factor), CH13_CH16_Rx/1(Factor), CH9_CH12_Rx/1(Factor), CH5_CH8_Rx/1(Factor)
  raptor_adjustment1/1 -> CH17_CH20_Rx1/2(Offset), CH13_CH16_Rx/2(Offset), CH9_CH12_Rx/2(Offset), CH5_CH8_Rx/2(Offset), CH1_CH4_Rx/2(Offset)

== system EPT/Foreground_TimeBase_5ms/CAN/CAN3_exec/DCDC ==
  Enable : EnablePort
  Constant1 : Constant  Value=20
  CountTrigger : Subsystem
  "DCDC_RX_0x180XF45D " : Subsystem  TreatAsAtomicUnit=on
  DCDC_TX_0x180XD5F4 : Subsystem  TreatAsAtomicUnit=on
  wires:
  Constant1/1 -> CountTrigger/1(Counter)
  CountTrigger/1(Tirgger) -> DCDC_TX_0x180XD5F4/Trigger, "DCDC_RX_0x180XF45D "/Trigger

== system EPT/Foreground_TimeBase_5ms/CAN/CAN3_exec/HyPer9_MCU ==
  Enable : EnablePort
  Constant2 : Constant  Value=4
  CountTrigger2 : Subsystem
  Delay : Delay  DelayLength=1
  Delay1 : Delay  DelayLength=1
  RPDO1 : Subsystem  TreatAsAtomicUnit=on
      settings: RTWSystemCode=Nonreusable function
  RPDO2 : Subsystem  TreatAsAtomicUnit=on
      settings: RTWSystemCode=Nonreusable function
  RPDO3 : Subsystem  TreatAsAtomicUnit=on
      settings: RTWSystemCode=Nonreusable function
  RPDO4 : Subsystem  TreatAsAtomicUnit=on
      settings: RTWSystemCode=Nonreusable function
  TPDO1 : Subsystem  TreatAsAtomicUnit=on
      settings: RTWSystemCode=Nonreusable function
  TPDO2 : Subsystem  TreatAsAtomicUnit=on
      settings: RTWSystemCode=Nonreusable function
  TPDO3 : Subsystem  TreatAsAtomicUnit=on
      settings: RTWSystemCode=Nonreusable function
  TPDO4 : Subsystem  TreatAsAtomicUnit=on
      settings: RTWSystemCode=Nonreusable function
  TPDO5 : Subsystem  TreatAsAtomicUnit=on
      settings: RTWSystemCode=Nonreusable function
  TPDO6 : Subsystem  TreatAsAtomicUnit=on
      settings: RTWSystemCode=Nonreusable function
  wires:
  Delay/1 -> Delay1/1, RPDO4/Trigger, TPDO4/Trigger, RPDO3/Trigger, TPDO3/Trigger
  Constant2/1 -> CountTrigger2/1(Counter)
  CountTrigger2/1(Tirgger) -> Delay/1, RPDO2/Trigger, TPDO2/Trigger, RPDO1/Trigger, TPDO1/Trigger
  Delay1/1 -> TPDO6/Trigger, TPDO5/Trigger

== system EPT/Foreground_TimeBase_5ms/CAN/CAN3_exec/OBC ==
  Enable : EnablePort
  CountTrigger : Subsystem
  CountTrigger1 : Subsystem
  OBC : Subsystem
  raptor_adjustment1 : Raptor_lib/Data Storage/raptor_adjustment  paramName='Cal_OBC_Rx_Time'  nameSource=Parameter  initValue=20  dataType=double  storage=Calibration  calDispType=Number  calEnum={'False', 'True'}  calGain=1.0  calOffset=0.0  calMax=inf  calMin=-inf  calFormat='-1'  calUnit=''  calHelp=''  calAccess=1  calFunction=raptor_xcp_function(gcb)  calDispHeaders=off  calColHeaders={'Col1' 'Col2' 'Col3'}  calRowHeaders={'Row1' 'Row2' 'Row3'}
      settings: SourceProductName=Raptor
  raptor_adjustment2 : Raptor_lib/Data Storage/raptor_adjustment  paramName='Cal_OBC_Tx_Time'  nameSource=Parameter  initValue=200  dataType=double  storage=Calibration  calDispType=Number  calEnum={'False', 'True'}  calGain=1.0  calOffset=0.0  calMax=inf  calMin=-inf  calFormat='-1'  calUnit=''  calHelp=''  calAccess=1  calFunction=raptor_xcp_function(gcb)  calDispHeaders=off  calColHeaders={'Col1' 'Col2' 'Col3'}  calRowHeaders={'Row1' 'Row2' 'Row3'}
      settings: SourceProductName=Raptor
  wires:
  CountTrigger1/1(Tirgger) -> OBC/1(Rx_Time)
  raptor_adjustment2/1 -> CountTrigger/1(Counter)
  CountTrigger/1(Tirgger) -> OBC/2(Tx_Time)
  raptor_adjustment1/1 -> CountTrigger1/1(Counter)

== system EPT/Foreground_TimeBase_5ms/CAN/CAN3_exec/PWCU_GENERATOR ==
  Enable : EnablePort
  CountTrigger : Subsystem
  CountTrigger1 : Subsystem
  PWCU : Subsystem
  raptor_adjustment1 : Raptor_lib/Data Storage/raptor_adjustment  paramName='Cal_PWCU_Rx_Time'  nameSource=Parameter  initValue=20  dataType=double  storage=Calibration  calDispType=Number  calEnum={'False', 'True'}  calGain=1.0  calOffset=0.0  calMax=inf  calMin=-inf  calFormat='-1'  calUnit=''  calHelp=''  calAccess=1  calFunction=raptor_xcp_function(gcb)  calDispHeaders=off  calColHeaders={'Col1' 'Col2' 'Col3'}  calRowHeaders={'Row1' 'Row2' 'Row3'}
      settings: SourceProductName=Raptor
  raptor_adjustment2 : Raptor_lib/Data Storage/raptor_adjustment  paramName='Cal_PWCU_Tx_Time'  nameSource=Parameter  initValue=200  dataType=double  storage=Calibration  calDispType=Number  calEnum={'False', 'True'}  calGain=1.0  calOffset=0.0  calMax=inf  calMin=-inf  calFormat='-1'  calUnit=''  calHelp=''  calAccess=1  calFunction=raptor_xcp_function(gcb)  calDispHeaders=off  calColHeaders={'Col1' 'Col2' 'Col3'}  calRowHeaders={'Row1' 'Row2' 'Row3'}
      settings: SourceProductName=Raptor
  wires:
  raptor_adjustment1/1 -> CountTrigger1/1(Counter)
  CountTrigger/1(Tirgger) -> PWCU/2(Tx_Time)
  raptor_adjustment2/1 -> CountTrigger/1(Counter)
  CountTrigger1/1(Tirgger) -> PWCU/1(Rx_Time)

== system EPT/Foreground_TimeBase_5ms/CAN/CAN3_exec/SEVCON_MCU  ==
  Enable : EnablePort
  Constant2 : Constant  Value=4
  Constant4 : Constant  Value=100
  CountTrigger1 : Subsystem
  CountTrigger2 : Subsystem
  Delay1 : Delay  DelayLength=1
  Delay2 : Delay  DelayLength=1
  SEVCON_Error_Code : Subsystem
  SEVCON_RX_0X220_20ms : Subsystem  TreatAsAtomicUnit=on
  SEVCON_RX_0X221_20ms : Subsystem  TreatAsAtomicUnit=on
  SEVCON_RX_0x701_500ms : Subsystem  TreatAsAtomicUnit=on
  "SEVCON_TX_0X210_20ms " : Subsystem  TreatAsAtomicUnit=on
  "SEVCON_TX_0X211_20ms " : Subsystem  TreatAsAtomicUnit=on
  wires:
  CountTrigger2/1(Tirgger) -> SEVCON_RX_0X220_20ms/Trigger, "SEVCON_TX_0X210_20ms "/Trigger, Delay1/1, Delay2/1
  CountTrigger1/1(Tirgger) -> SEVCON_RX_0x701_500ms/Trigger
  Constant4/1 -> CountTrigger1/1(Counter)
  Constant2/1 -> CountTrigger2/1(Counter)
  "SEVCON_TX_0X210_20ms "/1(Reverse) -> "SEVCON_TX_0X211_20ms "/1(Cmd_Reverse_Switch)
  "SEVCON_TX_0X210_20ms "/2(Forward) -> "SEVCON_TX_0X211_20ms "/2(Cmd_Forward_Switch)
  Delay1/1 -> "SEVCON_TX_0X211_20ms "/Trigger
  Delay2/1 -> SEVCON_RX_0X221_20ms/Trigger

== system EPT/Foreground_TimeBase_5ms/CAN/CAN3_exec/SWCU ==
  Enable : EnablePort
  Constant1 : Constant  Value=20
  Constant2 : Constant  Value=40
  CountTrigger : Subsystem
  CountTrigger1 : Subsystem
  Delay{,1..5} (6 alike) : Delay
  EPT to SWCU Enable Control : Subsystem  TreatAsAtomicUnit=on
  "SWCU OP Status-G1/G2 " : Subsystem  TreatAsAtomicUnit=on
  SWCU OP Status-G3 : Subsystem  TreatAsAtomicUnit=on
  "SWCU OP Status-G4 " : Subsystem  TreatAsAtomicUnit=on
  "SWCU OP Status-G5 " : Subsystem  TreatAsAtomicUnit=on
  SWCU OP Status-G6 : Subsystem  TreatAsAtomicUnit=on
  SWCU OP Status-G7 : Subsystem  TreatAsAtomicUnit=on
  SWCU OP Status-G8 : Subsystem  TreatAsAtomicUnit=on
  wires:
  Constant1/1 -> CountTrigger/1(Counter)
  CountTrigger/1(Tirgger) -> "SWCU OP Status-G1/G2 "/Trigger, Delay/1
  Constant2/1 -> CountTrigger1/1(Counter)
  Delay/1 -> EPT to SWCU Enable Control/Trigger
  CountTrigger1/1(Tirgger) -> Delay1/1, SWCU OP Status-G3/Trigger
  Delay1/1 -> Delay2/1, SWCU OP Status-G6/Trigger
  Delay2/1 -> Delay3/1, "SWCU OP Status-G4 "/Trigger
  Delay3/1 -> Delay4/1, SWCU OP Status-G7/Trigger
  Delay4/1 -> Delay5/1, "SWCU OP Status-G5 "/Trigger
  Delay5/1 -> SWCU OP Status-G8/Trigger

== system EPT/Foreground_TimeBase_5ms/CHG//DCHG_PW_Control/CHG//DCHG_Current_Control/Idchg_con Soft Recovery ==
  Idchg_con_input : Inport
  Add : Sum
  Constant : Constant
  Delay : Delay  DelayLength=1
  Delay1 : Subsystem
  Latch1 : Subsystem
  Logical Operator : Logic  Operator=OR  AllPortsSameDT=off  OutDataTypeStr=boolean
  NOT : Logic  Operator=NOT  IconShape=distinctive  AllPortsSameDT=off  OutDataTypeStr=boolean
  Relational Operator1 : RelationalOperator  Operator=>  OutDataTypeStr=boolean  RndMeth=Simplest
  Switch : Switch  Criteria=u2 > Threshold
      settings: LockScale=on
  raptor_adjustment1 : Raptor_lib/Data Storage/raptor_adjustment  paramName='Cal_Idschg_con_Soft_recovery_TimeCount'  nameSource=Parameter  initValue=800  dataType=double  storage=Calibration  calDispType=Number  calEnum={'False', 'True'}  calGain=1.0  calOffset=0.0  calMax=inf  calMin=-inf  calFormat='-1'  calUnit=''  calHelp=''  calAccess=1  calFunction=raptor_xcp_function(gcb)  calDispHeaders=off  calColHeaders={'Col1' 'Col2' 'Col3'}  calRowHeaders={'Row1' 'Row2' 'Row3'}
      settings: SourceProductName=Raptor
  raptor_adjustment2 : Raptor_lib/Data Storage/raptor_adjustment  paramName='Cal_Idschg_con_Soft_recovery_KI'  nameSource=Parameter  initValue=-0.001  dataType=double  storage=Calibration  calDispType=Number  calEnum={'False', 'True'}  calGain=1.0  calOffset=0.0  calMax=inf  calMin=-inf  calFormat='-1'  calUnit=''  calHelp=''  calAccess=1  calFunction=raptor_xcp_function(gcb)  calDispHeaders=off  calColHeaders={'Col1' 'Col2' 'Col3'}  calRowHeaders={'Row1' 'Row2' 'Row3'}
      settings: SourceProductName=Raptor
  Idchg_con_output : Outport
  wires:
  Idchg_con_input/1 -> Switch/1, Relational Operator1/1
  Delay/1 -> Add/1, Relational Operator1/2
  Relational Operator1/1 -> Logical Operator/1
  Constant/1 -> Delay1/1(Condition)
  Latch1/1(Output) -> NOT/1
  Logical Operator/1 -> Switch/2
  raptor_adjustment1/1 -> Delay1/2(TimeCount)
  Delay1/1(Output) -> Latch1/1(Latch)
  NOT/1 -> Logical Operator/2
  Switch/1 -> Idchg_con_output/1, Delay/1
  Add/1 -> Switch/3
  raptor_adjustment2/1 -> Add/2
